simulink model "PVAndBatteryIntegratedPlantForBlackStart"  (R2025b)
settings: Solver=FixedStepAuto  StartTime=0.0  StopTime=tsim  FixedStep=1e-6  RelTol=1e-9  AbsTol=1e-7
InitFcn:
  | %% Black Start Sequence
  | t0 = 0; % Battery IBR initial time
  | t1 = 0.15; % PV IBR initial time
  | t2 = 0.5; % Two IBR sync time
  | t3 = 0.8; % Additional motor load connect
  | t4 = 1.1; % Grid reconnection
  | tsim = 1.5; % Total simulation time
  | 
  | %% initialize
  | Vdc = 400;
  | Vnom = 100;
  | Prated = 10000;
  | Qrated = 0;
  | Srated = sqrt(Prated^2+Qrated^2);
  | wnom = 2*pi*60;
  | fnom = 60;
  | Vminpu = 0.95;
  | 
  | kv = Vnom;
  | ki = 3*Vnom/Srated;
  | 
  | dwmax = 0.5*2*pi;
  | trisemax = 0.1;
  | 
  | C = 1/sqrt(2)/Vminpu^2/dwmax;
  | L = 1/C/wnom^2;
  | tau = C/kv/ki;
  | epsilon = sqrt(L/C);
  | ksy = 3/2/trisemax;
  | 
  | V_voc_1 = 0;
  | V_voc_2 = 0;
  | 
  | % filter
  | Rf = 0.05;
  | Lf = 500e-6;
  | % pwm
  | fsw = 10e3;
  | % simulation
  | Ts = 1e-6;
  | 
  | % load
  | Rl = 3*Vnom^2/Prated;
  | Rl1 = Rl;
  | Rl2 = 2*Rl;
  | Rl3 = 20*Rl;
  | % grid
  | Rg = 0.05;
  | Lg = 50e-6;
  | 
  | % DCDC converter
  | Kp_V = 1;
  | Ki_V = 0.02;
  | Imax = 110;
  | Kp_I = 0.0001;
  | Ki_I = 1;
  | Vcmax = 1;
undefined symbols (not defined in the file): alpha, C_voc, Diode_class, Half_BridgeConverter_class, L_voc, Ll, Mosfet_class, PWMGenerator_DC_DC__class, R_voc, Three_PhaseBreaker_class, Three_PhaseSource_class, Three_PhaseTransformer_2_class, Three_PhaseV_IMeasuremen_class
libraries: nesl_utility x69, ee_lib x49, fl_lib x36, mcbeeMathTransformLib x9, simulink x6, spsParallelRLCBranchLib x3, eePwmGeneratorTwoLevel x2, spsControlledCurrentSourceLib x2, elec_conv_HighZElecRef x2, slpidlib x2, spsSecondOrderFilterLib x1, spsCurrentMeasurementLib x1
(part 4 of 4)

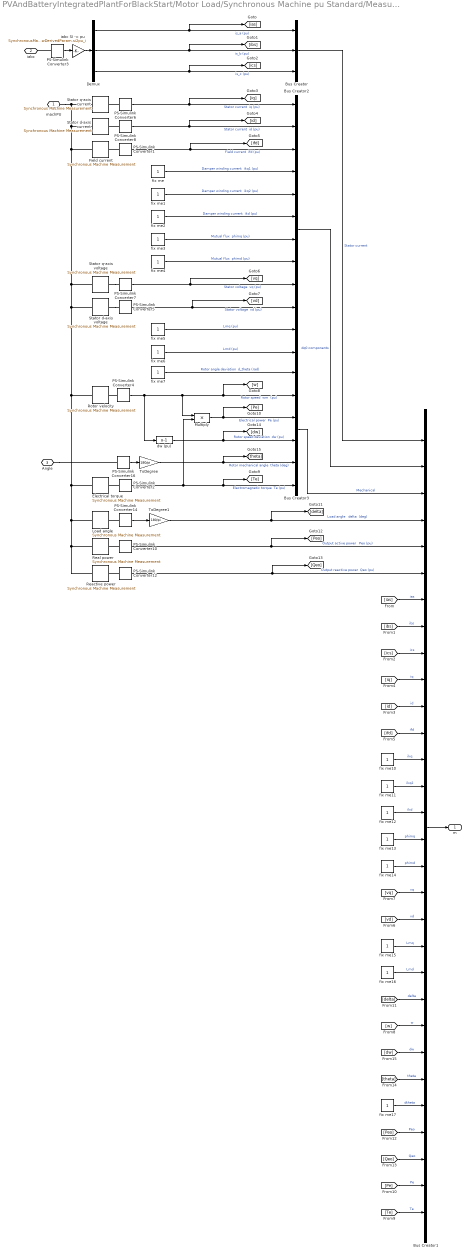
== system PVAndBatteryIntegratedPlantForBlackStart/Motor Load/Synchronous Machine pu Standard/Measurement ==
  Bus Creator : BusCreator  Inputs=3
  Bus Creator1 : BusCreator  Inputs=30
  Bus Creator2 : BusCreator  Inputs=12
  Bus Creator3 : BusCreator  Inputs=6
  Demux : Demux  Outputs=3
  Electrical torque : ee_lib/Electromechanical/Synchronous/Synchronous Machine Measurement  output_idx=3
      settings: InternalSimscapePortConfiguration="{\"Bottom\":[],\"Left\":[{\"id\":\"pu_input\",\"label\":\"pu\",\"type\":\"input\"}],\"Right\":[{\"id\":\"pu_output\",\"label\":\"o\",\"type\":\"output\"}],\"Top\":[]}"
  Field current : ee_lib/Electromechanical/Synchronous/Synchronous Machine Measurement  output_idx=2
      settings: InternalSimscapePortConfiguration="{\"Bottom\":[],\"Left\":[{\"id\":\"pu_input\",\"label\":\"pu\",\"type\":\"input\"}],\"Right\":[{\"id\":\"pu_output\",\"label\":\"o\",\"type\":\"output\"}],\"Top\":[]}"
  Load angle : ee_lib/Electromechanical/Synchronous/Synchronous Machine Measurement  output_idx=18
      settings: InternalSimscapePortConfiguration="{\"Bottom\":[],\"Left\":[{\"id\":\"pu_input\",\"label\":\"pu\",\"type\":\"input\"}],\"Right\":[{\"id\":\"pu_output\",\"label\":\"o\",\"type\":\"output\"}],\"Top\":[]}"
  Multiply : Product
  PS-Simulink Converter{1..8,10,12,14,16} (12 alike) : nesl_utility/PS-Simulink Converter  PhysicalDomain=network_engine_domain  SubClassName=ps_output  LeftPortType=input  RightPortType=output  PseudoPeriodic=off  Frequencies=[]  VectorFormat=1-D array  Unit=1  AffineConversion=off
  Reactive power : ee_lib/Electromechanical/Synchronous/Synchronous Machine Measurement  output_idx=13
      settings: InternalSimscapePortConfiguration="{\"Bottom\":[],\"Left\":[{\"id\":\"pu_input\",\"label\":\"pu\",\"type\":\"input\"}],\"Right\":[{\"id\":\"pu_output\",\"label\":\"o\",\"type\":\"output\"}],\"Top\":[]}"
  Real power : ee_lib/Electromechanical/Synchronous/Synchronous Machine Measurement  output_idx=12
      settings: InternalSimscapePortConfiguration="{\"Bottom\":[],\"Left\":[{\"id\":\"pu_input\",\"label\":\"pu\",\"type\":\"input\"}],\"Right\":[{\"id\":\"pu_output\",\"label\":\"o\",\"type\":\"output\"}],\"Top\":[]}"
  Rotor velocity : ee_lib/Electromechanical/Synchronous/Synchronous Machine Measurement  output_idx=4
      settings: InternalSimscapePortConfiguration="{\"Bottom\":[],\"Left\":[{\"id\":\"pu_input\",\"label\":\"pu\",\"type\":\"input\"}],\"Right\":[{\"id\":\"pu_output\",\"label\":\"o\",\"type\":\"output\"}],\"Top\":[]}"
  Stator d-axis current : ee_lib/Electromechanical/Synchronous/Synchronous Machine Measurement  output_idx=8
      settings: InternalSimscapePortConfiguration="{\"Bottom\":[],\"Left\":[{\"id\":\"pu_input\",\"label\":\"pu\",\"type\":\"input\"}],\"Right\":[{\"id\":\"pu_output\",\"label\":\"o\",\"type\":\"output\"}],\"Top\":[]}"
  Stator d-axis voltage : ee_lib/Electromechanical/Synchronous/Synchronous Machine Measurement  output_idx=5
      settings: InternalSimscapePortConfiguration="{\"Bottom\":[],\"Left\":[{\"id\":\"pu_input\",\"label\":\"pu\",\"type\":\"input\"}],\"Right\":[{\"id\":\"pu_output\",\"label\":\"o\",\"type\":\"output\"}],\"Top\":[]}"
  Stator q-axis current : ee_lib/Electromechanical/Synchronous/Synchronous Machine Measurement  output_idx=9
      settings: InternalSimscapePortConfiguration="{\"Bottom\":[],\"Left\":[{\"id\":\"pu_input\",\"label\":\"pu\",\"type\":\"input\"}],\"Right\":[{\"id\":\"pu_output\",\"label\":\"o\",\"type\":\"output\"}],\"Top\":[]}"
  Stator q-axis voltage : ee_lib/Electromechanical/Synchronous/Synchronous Machine Measurement  output_idx=6
      settings: InternalSimscapePortConfiguration="{\"Bottom\":[],\"Left\":[{\"id\":\"pu_input\",\"label\":\"pu\",\"type\":\"input\"}],\"Right\":[{\"id\":\"pu_output\",\"label\":\"o\",\"type\":\"output\"}],\"Top\":[]}"
  ToDegree : Gain  Gain=180/pi
  ToDegree1 : Gain  Gain=180/pi
  dw (pu) : Bias  Bias=-1  SaturateOnIntegerOverflow=off
  fix me{,1..7,10..17} (16 alike) : Constant
  "iabc SI -> pu" : Gain  Gain=SynchronousMachinePuStan_class('Mechanical power Pm',[6000 122.5 60],[0.1028 0.02056 2],20,[0 0 0 0 0 0 0 0 1],[0.6404 0.7127 0.8441 0.9214 0.9956 1.082 1.19 1.316 1.457;0.7 0.7698 0.8872 0.9466 0.9969 1.046 1.1 1.151 1.201],'on','Salient-pole','Short-circuit','Short-circuit',[1.81 0.3 0.23 1.76 0.65 0.25 0.15],[2.24 0.17 0.12 1.02 0.13 0.08],[4.4849 0.0681 0.1],[8 0.03 1 0.07],[4.49 0.0681 0.0513],[8 0.03 0.3371 0.0295],[1.01 0.053 0.1],[1.3201 0.023 1 0.07],[0.012 0.003 0.003],[1.3201 0.0231 0.3371 0.0295]).objParamMappingDerived.NewDerivedParam.si2pu_i
  machPU : PMIOPort  Side=Left
  iabc : PMIOPort  Port=2  Side=Left
  Angle : PMIOPort  Port=3  Side=Left
  m : Outport  VectorParamsAs1DForOutWhenUnconnected=off
  wires:
  "iabc SI -> pu"/1 -> Demux/1
  PS-Simulink Converter12/1 -> Bus Creator1/6, [Qeo]  "Output reactive power  Qeo (pu)"
  PS-Simulink Converter10/1 -> Bus Creator1/5, [Peo]  "Output active power   Peo (pu)"
  PS-Simulink Converter14/1 -> ToDegree1/1
  PS-Simulink Converter3/1 -> "iabc SI -> pu"/1
  Demux/3 -> [ics], Bus Creator/3  "is_c (pu)"
  Demux/2 -> [ibs], Bus Creator/2  "is_b (pu)"
  Demux/1 -> [ias], Bus Creator/1  "is_a (pu)"
  Bus Creator3/1 -> Bus Creator1/3  "Mechanical"
  Bus Creator2/1 -> Bus Creator1/2  "dq0 components"
  Bus Creator/1 -> Bus Creator1/1  "Stator current"
  Bus Creator1/1 -> m/1
  PS-Simulink Converter8/1 -> [id], Bus Creator2/2  "Stator current  id (pu)"
  PS-Simulink Converter6/1 -> [iq], Bus Creator2/1  "Stator current  iq (pu)"
  PS-Simulink Converter5/1 -> Bus Creator2/10, [vd]  "Stator voltage  vd (pu)"
  PS-Simulink Converter7/1 -> Bus Creator2/9, [vq]  "Stator voltage  vq (pu)"
  PS-Simulink Converter4/1 -> dw (pu)/1, Bus Creator3/2, [w], Multiply/1  "Rotor speed  wm  (pu)"
  PS-Simulink Converter2/1 -> Multiply/2, [Te], Bus Creator3/6  "Electromagnetic torque  Te (pu)"
  PS-Simulink Converter1/1 -> [ifd], Bus Creator2/3  "Field current  ifd (pu)"
  Multiply/1 -> [Pe], Bus Creator3/3  "Electrical power  Pe (pu)"
  [ias] -> Bus Creator1/7  "ias"
  [ibs] -> Bus Creator1/8  "ibs"
  [ics] -> Bus Creator1/9  "ics"
  [ifd] -> Bus Creator1/12  "ifd"
  fix me6/1 -> Bus Creator2/12  "Lmd (pu)"
  fix me5/1 -> Bus Creator2/11  "Lmq (pu)"
  fix me7/1 -> Bus Creator3/1  "Rotor angle deviation  d_theta (rad)"
  dw (pu)/1 -> [dw], Bus Creator3/4  "Rotor speed deviation  dw (pu)"
  ToDegree/1 -> [theta], Bus Creator3/5  "Rotor mechanical angle  theta (deg)"
  PS-Simulink Converter16/1 -> ToDegree/1
  ToDegree1/1 -> Bus Creator1/4, [delta]  "Load angle   delta  (deg)"
  [id] -> Bus Creator1/11  "id"
  [iq] -> Bus Creator1/10  "iq"
  fix me10/1 -> Bus Creator1/13  "ikq"
  fix me11/1 -> Bus Creator1/14  "ikq2"
  fix me12/1 -> Bus Creator1/15  "ikd"
  fix me13/1 -> Bus Creator1/16  "phimq"
  fix me14/1 -> Bus Creator1/17  "phimd"
  [vq] -> Bus Creator1/18  "vq"
  [vd] -> Bus Creator1/19  "vd"
  fix me16/1 -> Bus Creator1/21  "Lmd"
  fix me15/1 -> Bus Creator1/20  "Lmq"
  [delta] -> Bus Creator1/22  "delta"
  [w] -> Bus Creator1/23  "w"
  [dw] -> Bus Creator1/24  "dw"
  [theta] -> Bus Creator1/25  "theta"
  fix me17/1 -> Bus Creator1/26  "dtheta"
  [Peo] -> Bus Creator1/27  "Peo"
  [Qeo] -> Bus Creator1/28  "Qeo"
  [Pe] -> Bus Creator1/29  "Pe"
  [Te] -> Bus Creator1/30  "Te"
  fix me/1 -> Bus Creator2/4  "Damper winding current  ikq1 (pu)"
  fix me1/1 -> Bus Creator2/5  "Damper winding current  ikq2 (pu)"
  fix me2/1 -> Bus Creator2/6  "Damper winding current  ikd (pu)"
  fix me3/1 -> Bus Creator2/7  "Mutual flux  phimq (pu)"
  fix me4/1 -> Bus Creator2/8  "Mutual flux  phimd (pu)"
  connections:
  PS-Simulink Converter3/LConn1 -- iabc/RConn1
  Stator q-axis current/LConn1 -- Stator d-axis voltage/LConn1 -- Reactive power/LConn1 -- Real power/LConn1 -- Load angle/LConn1 -- Electrical torque/LConn1 -- Rotor velocity/LConn1 -- Stator q-axis voltage/LConn1 -- Field current/LConn1 -- Stator d-axis current/LConn1 -- machPU/RConn1
  PS-Simulink Converter14/LConn1 -- Load angle/RConn1
  PS-Simulink Converter12/LConn1 -- Reactive power/RConn1
  PS-Simulink Converter10/LConn1 -- Real power/RConn1
  PS-Simulink Converter8/LConn1 -- Stator d-axis current/RConn1
  Stator d-axis voltage/RConn1 -- PS-Simulink Converter5/LConn1
  PS-Simulink Converter6/LConn1 -- Stator q-axis current/RConn1
  Stator q-axis voltage/RConn1 -- PS-Simulink Converter7/LConn1
  PS-Simulink Converter4/LConn1 -- Rotor velocity/RConn1
  PS-Simulink Converter2/LConn1 -- Electrical torque/RConn1
  PS-Simulink Converter1/LConn1 -- Field current/RConn1
  Angle/RConn1 -- PS-Simulink Converter16/LConn1

== system PVAndBatteryIntegratedPlantForBlackStart/PV Inverter /Inverter/Half-Bridge Converter ==
  " g " : Inport
  BL : Inport  Port=2
  Compare To Constant : simulink/Logic and Bit Operations/Compare To Constant  relop=<=  const=0.5  OutDataTypeStr=boolean
  Data Type Conversion : DataTypeConversion  OutDataTypeStr=double  SaturateOnIntegerOverflow=off  RndMeth=Floor
  Demux : Demux  Outputs=2
  Multiply : Product
  Simulink-PS Converter : nesl_utility/Simulink-PS Converter  PhysicalDomain=network_engine_domain  SubClassName=ps_input  LeftPortType=input  RightPortType=output  PseudoPeriodic=off  Frequencies=[]  NoiseDistribution=none  NoiseParameters=[]  Unit=1  AffineConversion=off  FilteringAndDerivatives=provide  SimscapeFilterOrder=1  InputFilterTimeConstant=0.001  UdotUserProvided=0
  Simulink-PS Converter1 : nesl_utility/Simulink-PS Converter  PhysicalDomain=network_engine_domain  SubClassName=ps_input  LeftPortType=input  RightPortType=output  PseudoPeriodic=off  Frequencies=[]  NoiseDistribution=none  NoiseParameters=[]  Unit=1  AffineConversion=off  FilteringAndDerivatives=provide  SimscapeFilterOrder=1  InputFilterTimeConstant=0.001  UdotUserProvided=0
  Two-Pulse Gate Multiplexer : ee_lib/Semiconductors & Converters/Converters/Two-Pulse Gate Multiplexer  port_option=ee.enum.controlport.ps
      settings: InternalSimscapePortConfiguration="{\"Bottom\":[],\"Left\":[{\"id\":\"G1_ps\",\"label\":\"G1\",\"type\":\"input\"},{\"id\":\"G2_ps\",\"label\":\"G2\",\"type\":\"input\"}],\"Right\":[{\"id\":\"p\",\"label\":\"G\",\"type\":\"foundation.electrical.four_phase\"}],\"Top\":[]}"
  Two-Quadrant Chopper : ee_lib/Semiconductors & Converters/Converters/Two-Quadrant Chopper  device_type=3  Vf=Half_BridgeConverter_class('Switching devices',0.001,1000000,Inf,0.001,1000000,Inf,0.001).objParamMappingDerived.NewDerivedParam.Vf V  Ron=Half_BridgeConverter_class('Switching devices',0.001,1000000,Inf,0.001,1000000,Inf,0.001).objParamMappingDerived.NewDerivedParam.Ron Ohm  Rds=0.001 Ohm  Goff=Half_BridgeConverter_class('Switching devices',0.001,1000000,Inf,0.001,1000000,Inf,0.001).objParamMappingDerived.NewDerivedParam.Goff 1/Ohm  Vgt=1 V  Vgt_off=-1 V  Ih=1 A  Vth=0.5 V  K=0  diode_param=2  diode_Vf=Half_BridgeConverter_class('Switching devices',0.001,1000000,Inf,0.001,1000000,Inf,0.001).objParamMappingDerived.NewDerivedParam.diode_Vf V  diode_Ron=Half_BridgeConverter_class('Switching devices',0.001,1000000,Inf,0.001,1000000,Inf,0.001).objParamMappingDerived.NewDerivedParam.diode_Ron Ohm  diode_Goff=Half_BridgeConverter_class('Switching devices',0.001,1000000,Inf,0.001,1000000,Inf,0.001).objParamMappingDerived.NewDerivedParam.diode_Goff 1/Ohm  diode_C=50 nF  diode_iRM=-235 A  diode_iF=300 A  diode_idot=-50 A/us  diode_trr_param=1  diode_trr_factor=3  diode_trr=15 us  diode_Qrr=1500 s*uA  snubber_type=0  Cs=Half_BridgeConverter_class('Switching devices',0.001,1000000,Inf,0.001,1000000,Inf,0.001).objParamMappingDerived.NewDerivedParam.Cs F  Rs=Half_BridgeConverter_class('Switching devices',0.001,1000000,Inf,0.001,1000000,Inf,0.001).objParamMappingDerived.NewDerivedParam.Rs Ohm
      settings: InternalSimscapePortConfiguration="{\"Bottom\":[],\"Left\":[{\"id\":\"G\",\"label\":\"G\",\"type\":\"foundation.electrical.four_phase\"},{\"id\":\"p1\",\"label\":\"1+\",\"type\":\"foundation.electrical.electrical\"},{\"id\":\"n1\",\"label\":\"1-\",\"type\":\"foundation.electrical.electrical\"}],\"Right\":[{\"id\":\"p2\",\"label\":\"2+\",\"type\":\"foundation.electrical.electrical\"},{\"id\":\"n2\",\"label\":\"2-\",\"type\":\"foundation.electrical.electrical\"}],\"Top\":[]}"
  + : PMIOPort  Side=Right
  - : PMIOPort  Port=2  Side=Right
  1 : PMIOPort  Port=3  Side=Left
  wires:
  Demux/2 -> Simulink-PS Converter1/1
  Demux/1 -> Simulink-PS Converter/1
  Multiply/1 -> Demux/1
  Data Type Conversion/1 -> Multiply/2
  Compare To Constant/1 -> Data Type Conversion/1
  BL/1 -> Compare To Constant/1
  " g "/1 -> Multiply/1
  connections:
  Simulink-PS Converter1/RConn1 -- Two-Pulse Gate Multiplexer/LConn2
  Two-Pulse Gate Multiplexer/RConn1 -- Two-Quadrant Chopper/LConn1
  Simulink-PS Converter/RConn1 -- Two-Pulse Gate Multiplexer/LConn1
  +/RConn1 -- Two-Quadrant Chopper/LConn2
  1/RConn1 -- Two-Quadrant Chopper/RConn1
  Two-Quadrant Chopper/LConn3 -- Two-Quadrant Chopper/RConn2 -- -/RConn1

== system PVAndBatteryIntegratedPlantForBlackStart/PV Inverter /Inverter/Half-Bridge Converter1 ==
  " g " : Inport
  BL : Inport  Port=2
  Compare To Constant : simulink/Logic and Bit Operations/Compare To Constant  relop=<=  const=0.5  OutDataTypeStr=boolean
  Data Type Conversion : DataTypeConversion  OutDataTypeStr=double  SaturateOnIntegerOverflow=off  RndMeth=Floor
  Demux : Demux  Outputs=2
  Multiply : Product
  Simulink-PS Converter : nesl_utility/Simulink-PS Converter  PhysicalDomain=network_engine_domain  SubClassName=ps_input  LeftPortType=input  RightPortType=output  PseudoPeriodic=off  Frequencies=[]  NoiseDistribution=none  NoiseParameters=[]  Unit=1  AffineConversion=off  FilteringAndDerivatives=provide  SimscapeFilterOrder=1  InputFilterTimeConstant=0.001  UdotUserProvided=0
  Simulink-PS Converter1 : nesl_utility/Simulink-PS Converter  PhysicalDomain=network_engine_domain  SubClassName=ps_input  LeftPortType=input  RightPortType=output  PseudoPeriodic=off  Frequencies=[]  NoiseDistribution=none  NoiseParameters=[]  Unit=1  AffineConversion=off  FilteringAndDerivatives=provide  SimscapeFilterOrder=1  InputFilterTimeConstant=0.001  UdotUserProvided=0
  Two-Pulse Gate Multiplexer : ee_lib/Semiconductors & Converters/Converters/Two-Pulse Gate Multiplexer  port_option=ee.enum.controlport.ps
      settings: InternalSimscapePortConfiguration="{\"Bottom\":[],\"Left\":[{\"id\":\"G1_ps\",\"label\":\"G1\",\"type\":\"input\"},{\"id\":\"G2_ps\",\"label\":\"G2\",\"type\":\"input\"}],\"Right\":[{\"id\":\"p\",\"label\":\"G\",\"type\":\"foundation.electrical.four_phase\"}],\"Top\":[]}"
  Two-Quadrant Chopper : ee_lib/Semiconductors & Converters/Converters/Two-Quadrant Chopper  device_type=3  Vf=Half_BridgeConverter_class('Switching devices',0.001,1000000,Inf,0.001,1000000,Inf,0.001).objParamMappingDerived.NewDerivedParam.Vf V  Ron=Half_BridgeConverter_class('Switching devices',0.001,1000000,Inf,0.001,1000000,Inf,0.001).objParamMappingDerived.NewDerivedParam.Ron Ohm  Rds=0.001 Ohm  Goff=Half_BridgeConverter_class('Switching devices',0.001,1000000,Inf,0.001,1000000,Inf,0.001).objParamMappingDerived.NewDerivedParam.Goff 1/Ohm  Vgt=1 V  Vgt_off=-1 V  Ih=1 A  Vth=0.5 V  K=0  diode_param=2  diode_Vf=Half_BridgeConverter_class('Switching devices',0.001,1000000,Inf,0.001,1000000,Inf,0.001).objParamMappingDerived.NewDerivedParam.diode_Vf V  diode_Ron=Half_BridgeConverter_class('Switching devices',0.001,1000000,Inf,0.001,1000000,Inf,0.001).objParamMappingDerived.NewDerivedParam.diode_Ron Ohm  diode_Goff=Half_BridgeConverter_class('Switching devices',0.001,1000000,Inf,0.001,1000000,Inf,0.001).objParamMappingDerived.NewDerivedParam.diode_Goff 1/Ohm  diode_C=50 nF  diode_iRM=-235 A  diode_iF=300 A  diode_idot=-50 A/us  diode_trr_param=1  diode_trr_factor=3  diode_trr=15 us  diode_Qrr=1500 s*uA  snubber_type=0  Cs=Half_BridgeConverter_class('Switching devices',0.001,1000000,Inf,0.001,1000000,Inf,0.001).objParamMappingDerived.NewDerivedParam.Cs F  Rs=Half_BridgeConverter_class('Switching devices',0.001,1000000,Inf,0.001,1000000,Inf,0.001).objParamMappingDerived.NewDerivedParam.Rs Ohm
      settings: InternalSimscapePortConfiguration="{\"Bottom\":[],\"Left\":[{\"id\":\"G\",\"label\":\"G\",\"type\":\"foundation.electrical.four_phase\"},{\"id\":\"p1\",\"label\":\"1+\",\"type\":\"foundation.electrical.electrical\"},{\"id\":\"n1\",\"label\":\"1-\",\"type\":\"foundation.electrical.electrical\"}],\"Right\":[{\"id\":\"p2\",\"label\":\"2+\",\"type\":\"foundation.electrical.electrical\"},{\"id\":\"n2\",\"label\":\"2-\",\"type\":\"foundation.electrical.electrical\"}],\"Top\":[]}"
  + : PMIOPort  Side=Right
  - : PMIOPort  Port=2  Side=Right
  1 : PMIOPort  Port=3  Side=Left
  wires:
  Demux/2 -> Simulink-PS Converter1/1
  Demux/1 -> Simulink-PS Converter/1
  Multiply/1 -> Demux/1
  Data Type Conversion/1 -> Multiply/2
  Compare To Constant/1 -> Data Type Conversion/1
  BL/1 -> Compare To Constant/1
  " g "/1 -> Multiply/1
  connections:
  Simulink-PS Converter1/RConn1 -- Two-Pulse Gate Multiplexer/LConn2
  Two-Pulse Gate Multiplexer/RConn1 -- Two-Quadrant Chopper/LConn1
  Simulink-PS Converter/RConn1 -- Two-Pulse Gate Multiplexer/LConn1
  +/RConn1 -- Two-Quadrant Chopper/LConn2
  1/RConn1 -- Two-Quadrant Chopper/RConn1
  Two-Quadrant Chopper/LConn3 -- Two-Quadrant Chopper/RConn2 -- -/RConn1

== system PVAndBatteryIntegratedPlantForBlackStart/PV Inverter /Inverter/Half-Bridge Converter2 ==
  " g " : Inport
  BL : Inport  Port=2
  Compare To Constant : simulink/Logic and Bit Operations/Compare To Constant  relop=<=  const=0.5  OutDataTypeStr=boolean
  Data Type Conversion : DataTypeConversion  OutDataTypeStr=double  SaturateOnIntegerOverflow=off  RndMeth=Floor
  Demux : Demux  Outputs=2
  Multiply : Product
  Simulink-PS Converter : nesl_utility/Simulink-PS Converter  PhysicalDomain=network_engine_domain  SubClassName=ps_input  LeftPortType=input  RightPortType=output  PseudoPeriodic=off  Frequencies=[]  NoiseDistribution=none  NoiseParameters=[]  Unit=1  AffineConversion=off  FilteringAndDerivatives=provide  SimscapeFilterOrder=1  InputFilterTimeConstant=0.001  UdotUserProvided=0
  Simulink-PS Converter1 : nesl_utility/Simulink-PS Converter  PhysicalDomain=network_engine_domain  SubClassName=ps_input  LeftPortType=input  RightPortType=output  PseudoPeriodic=off  Frequencies=[]  NoiseDistribution=none  NoiseParameters=[]  Unit=1  AffineConversion=off  FilteringAndDerivatives=provide  SimscapeFilterOrder=1  InputFilterTimeConstant=0.001  UdotUserProvided=0
  Two-Pulse Gate Multiplexer : ee_lib/Semiconductors & Converters/Converters/Two-Pulse Gate Multiplexer  port_option=ee.enum.controlport.ps
      settings: InternalSimscapePortConfiguration="{\"Bottom\":[],\"Left\":[{\"id\":\"G1_ps\",\"label\":\"G1\",\"type\":\"input\"},{\"id\":\"G2_ps\",\"label\":\"G2\",\"type\":\"input\"}],\"Right\":[{\"id\":\"p\",\"label\":\"G\",\"type\":\"foundation.electrical.four_phase\"}],\"Top\":[]}"
  Two-Quadrant Chopper : ee_lib/Semiconductors & Converters/Converters/Two-Quadrant Chopper  device_type=3  Vf=Half_BridgeConverter_class('Switching devices',0.001,1000000,Inf,0.001,1000000,Inf,0.001).objParamMappingDerived.NewDerivedParam.Vf V  Ron=Half_BridgeConverter_class('Switching devices',0.001,1000000,Inf,0.001,1000000,Inf,0.001).objParamMappingDerived.NewDerivedParam.Ron Ohm  Rds=0.001 Ohm  Goff=Half_BridgeConverter_class('Switching devices',0.001,1000000,Inf,0.001,1000000,Inf,0.001).objParamMappingDerived.NewDerivedParam.Goff 1/Ohm  Vgt=1 V  Vgt_off=-1 V  Ih=1 A  Vth=0.5 V  K=0  diode_param=2  diode_Vf=Half_BridgeConverter_class('Switching devices',0.001,1000000,Inf,0.001,1000000,Inf,0.001).objParamMappingDerived.NewDerivedParam.diode_Vf V  diode_Ron=Half_BridgeConverter_class('Switching devices',0.001,1000000,Inf,0.001,1000000,Inf,0.001).objParamMappingDerived.NewDerivedParam.diode_Ron Ohm  diode_Goff=Half_BridgeConverter_class('Switching devices',0.001,1000000,Inf,0.001,1000000,Inf,0.001).objParamMappingDerived.NewDerivedParam.diode_Goff 1/Ohm  diode_C=50 nF  diode_iRM=-235 A  diode_iF=300 A  diode_idot=-50 A/us  diode_trr_param=1  diode_trr_factor=3  diode_trr=15 us  diode_Qrr=1500 s*uA  snubber_type=0  Cs=Half_BridgeConverter_class('Switching devices',0.001,1000000,Inf,0.001,1000000,Inf,0.001).objParamMappingDerived.NewDerivedParam.Cs F  Rs=Half_BridgeConverter_class('Switching devices',0.001,1000000,Inf,0.001,1000000,Inf,0.001).objParamMappingDerived.NewDerivedParam.Rs Ohm
      settings: InternalSimscapePortConfiguration="{\"Bottom\":[],\"Left\":[{\"id\":\"G\",\"label\":\"G\",\"type\":\"foundation.electrical.four_phase\"},{\"id\":\"p1\",\"label\":\"1+\",\"type\":\"foundation.electrical.electrical\"},{\"id\":\"n1\",\"label\":\"1-\",\"type\":\"foundation.electrical.electrical\"}],\"Right\":[{\"id\":\"p2\",\"label\":\"2+\",\"type\":\"foundation.electrical.electrical\"},{\"id\":\"n2\",\"label\":\"2-\",\"type\":\"foundation.electrical.electrical\"}],\"Top\":[]}"
  + : PMIOPort  Side=Right
  - : PMIOPort  Port=2  Side=Right
  1 : PMIOPort  Port=3  Side=Left
  wires:
  Demux/2 -> Simulink-PS Converter1/1
  Demux/1 -> Simulink-PS Converter/1
  Multiply/1 -> Demux/1
  Data Type Conversion/1 -> Multiply/2
  Compare To Constant/1 -> Data Type Conversion/1
  BL/1 -> Compare To Constant/1
  " g "/1 -> Multiply/1
  connections:
  Simulink-PS Converter1/RConn1 -- Two-Pulse Gate Multiplexer/LConn2
  Two-Pulse Gate Multiplexer/RConn1 -- Two-Quadrant Chopper/LConn1
  Simulink-PS Converter/RConn1 -- Two-Pulse Gate Multiplexer/LConn1
  +/RConn1 -- Two-Quadrant Chopper/LConn2
  1/RConn1 -- Two-Quadrant Chopper/RConn1
  Two-Quadrant Chopper/LConn3 -- Two-Quadrant Chopper/RConn2 -- -/RConn1

== system PVAndBatteryIntegratedPlantForBlackStart/PV Inverter /Three-Phase Breaker/com ==
  AND : Logic  Operator=NXOR  Inputs=5  IconShape=distinctive  AllPortsSameDT=off  OutDataTypeStr=boolean
  Data Type Conversion : DataTypeConversion  SaturateOnIntegerOverflow=off  RndMeth=Floor
  Simulink-PS Converter : nesl_utility/Simulink-PS Converter  PhysicalDomain=network_engine_domain  SubClassName=ps_input  LeftPortType=input  RightPortType=output  PseudoPeriodic=off  Frequencies=[]  NoiseDistribution=none  NoiseParameters=[]  Unit=1  AffineConversion=off  FilteringAndDerivatives=provide  SimscapeFilterOrder=1  InputFilterTimeConstant=0.001  UdotUserProvided=0
  Step : Step  Time=Three_PhaseBreaker_class('open',1000000,Inf,t1,'off').objParamMappingDerived.NewDerivedParam.switchTime1  SampleTime=0
  Step1 : Step  Time=Three_PhaseBreaker_class('open',1000000,Inf,t1,'off').objParamMappingDerived.NewDerivedParam.switchTime2  SampleTime=0
  Step2 : Step  Time=Three_PhaseBreaker_class('open',1000000,Inf,t1,'off').objParamMappingDerived.NewDerivedParam.switchTime3  SampleTime=0
  Step3 : Step  Time=Three_PhaseBreaker_class('open',1000000,Inf,t1,'off').objParamMappingDerived.NewDerivedParam.switchTime4  SampleTime=0
  Step4 : Step  Time=Three_PhaseBreaker_class('open',1000000,Inf,t1,'off').objParamMappingDerived.NewDerivedParam.switchTime5  SampleTime=0
  CB : PMIOPort  Side=Right
  wires:
  Data Type Conversion/1 -> Simulink-PS Converter/1
  Step4/1 -> AND/5
  AND/1 -> Data Type Conversion/1
  Step3/1 -> AND/4
  Step1/1 -> AND/2
  Step/1 -> AND/1
  Step2/1 -> AND/3
  connections:
  Simulink-PS Converter/RConn1 -- CB/RConn1

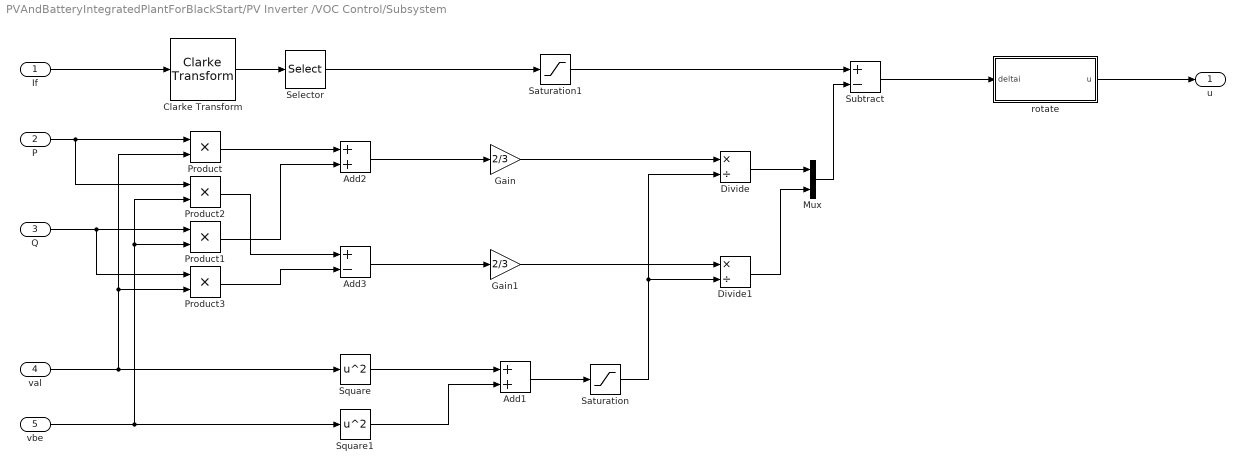
== system PVAndBatteryIntegratedPlantForBlackStart/PV Inverter /VOC Control/Subsystem ==
  If : Inport
  P : Inport  Port=2
  Q : Inport  Port=3
  val : Inport  Port=4
  vbe : Inport  Port=5
  Add1 : Sum
  Add2 : Sum
  Add3 : Sum  Inputs=+-
  Clarke Transform : mcbeeMathTransformLib/Clarke Transform  PowerInvariant=off  UseWithEmbedded=off  PhaseInput=Two inputs
      settings: LibrarySourceBlock=|
      | ee_sl_lib/Mathematical
      | Transforms/Clarke Transform
  Divide : Product  Inputs=*/
  Divide1 : Product  Inputs=*/
  Gain : Gain  Gain=2/3
  Gain1 : Gain  Gain=2/3
  Mux : Mux  Inputs=2
  Product{,1..3} (4 alike) : Product
  Saturation : Saturate  UpperLimit=inf  LowerLimit=1e-9
  Saturation1 : Saturate  UpperLimit=1e3  LowerLimit=-1e3
  Selector : Selector  InputPortWidth=3  IndexOptions=Index vector (dialog)  Indices=[1 2]  OutputSizes=1
  Square : Math  Operator=square
  Square1 : Math  Operator=square
  Subtract : Sum  Inputs=+-
  rotate : Subsystem
  u : Outport
  wires:
  rotate/1(u) -> u/1
  Subtract/1 -> rotate/1(deltai)
  Mux/1 -> Subtract/2
  Divide1/1 -> Mux/2
  Divide/1 -> Mux/1
  Gain1/1 -> Divide1/1
  Add3/1 -> Gain1/1
  Product3/1 -> Add3/2
  Product2/1 -> Add3/1
  Saturation/1 -> Divide1/2, Divide/2
  Gain/1 -> Divide/1
  Add2/1 -> Gain/1
  Product1/1 -> Add2/2
  Product/1 -> Add2/1
  Q/1 -> Product1/1, Product3/1
  P/1 -> Product/1, Product2/1
  Add1/1 -> Saturation/1
  Square1/1 -> Add1/2
  Square/1 -> Add1/1
  vbe/1 -> Square1/1, Product1/2, Product2/2
  val/1 -> Square/1, Product/2, Product3/2
  If/1 -> Clarke Transform/1
  Clarke Transform/1 -> Selector/1
  Selector/1 -> Saturation1/1
  Saturation1/1 -> Subtract/1

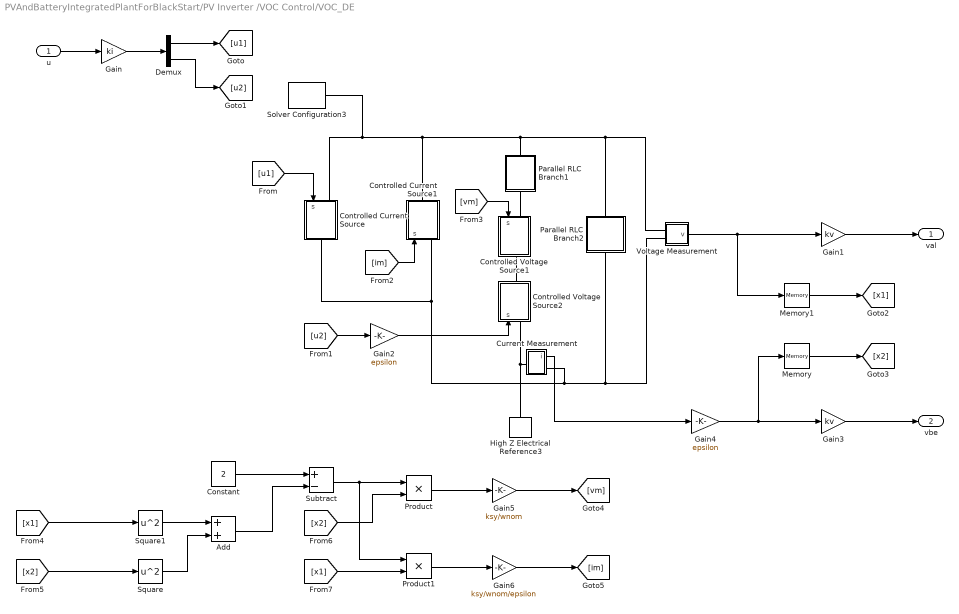
== system PVAndBatteryIntegratedPlantForBlackStart/PV Inverter /VOC Control/VOC_DE ==
  u : Inport
  Add : Sum
  Constant : Constant  Value=2
  Controlled Current Source : Subsystem
      settings: OpenFcn=elec.conv.unmask(gcb);
  Controlled Current Source1 : Subsystem
      settings: OpenFcn=elec.conv.unmask(gcb);
  Controlled Voltage Source1 : Subsystem
      settings: OpenFcn=elec.conv.unmask(gcb);
  Controlled Voltage Source2 : Subsystem
      settings: OpenFcn=elec.conv.unmask(gcb);
  Current Measurement : Subsystem
      settings: OpenFcn=elec.conv.unmask(gcb);
  Demux : Demux  Outputs=2
  Gain : Gain  Gain=ki
  Gain1 : Gain  Gain=kv
  Gain2 : Gain  Gain=epsilon
  Gain3 : Gain  Gain=kv
  Gain4 : Gain  Gain=epsilon
  Gain5 : Gain  Gain=ksy/wnom
  Gain6 : Gain  Gain=ksy/wnom/epsilon
  High Z Electrical Reference3 : elec_conv_HighZElecRef/High Z Electrical Reference  SystemSampleTime=-1  VariantActivationTime=update diagram  EmptyChoice=off  PassThrough=off  PassThroughVariantControl=(default)  EmptyChoiceVariantControl=(default)  AllowFlexibleInterface=on  Latency=0  AutoFrameSizeCalculation=off
  Memory : Memory
  Memory1 : Memory
  Parallel RLC Branch1 : Subsystem
      settings: AttributesFormatString=\n  OpenFcn=elec.conv.unmask(gcb);
  Parallel RLC Branch2 : Subsystem
      settings: AttributesFormatString=\n  OpenFcn=elec.conv.unmask(gcb);
  Product : Product
  Product1 : Product
  Solver Configuration3 : nesl_utility/Solver Configuration  PhysicalDomain=network_engine_domain  SubClassName=solver  LeftPortType=input  RightPortType=generic  Tones=[]  Harmonics=[]  SimulateNoise=off  Profile=off  UseLocalSampling=off  EnableSwitchedLinearOptims=on  FrequencyDomain=off  UseCCode=off  RelTol=0.001  AbsTol=0.001  MinStep=1e-09  ToWorkspace=off  RevertToSquareIcSolve=off  NumHomotopyIterations=100  PhasorMode=off  PhasorModeNumHarmonics=1  ConsistencySolver=NEWTON_XTOL_AFTER_FTOL  IndexReductionMethod=DerivativeReplacement  DoDC=off  ResidualTolerance=1e-09  ConsistencyTolSource=GLOBAL  ConsistencyAbsTol=0.001  ConsistencyRelTol=0.001  ConsistencyTolFactor=0.001  UseLocalSolver=off  LocalSolverChoice=NE_BACKWARD_EULER_ADVANCER  ResolveIndetEquations=on  FunctionEvalNumThread=1  LocalSolverSampleTime=1e-6  DoFixedCost=on  MaxNonlinIter=3  MaxModeIter=2  ComputeImpulses=off  ImpulseIterations=2  LinearAlgebra=auto  LinearAlgebraNumThread=0  EquationFormulation=NE_TIME_EF  DelaysMemoryBudget=1024  AutomaticFiltering=on  FilteringTimeConstant=0.001  PartitionStorageMethod=AS_NEEDED  PartitionMemoryBudget=1024  PartitionMethod=ROBUST  MultibodyUseLocalSolver=off  MultibodyLocalSolverChoice=ODE1  MultibodyLocalSolverSampleTime=0.001
  Square : Math  Operator=square
  Square1 : Math  Operator=square
  Subtract : Sum  Inputs=+-
  Voltage Measurement : Subsystem
      settings: OpenFcn=elec.conv.unmask(gcb);
  val : Outport
  vbe : Outport  Port=2
  wires:
  Gain6/1 -> [im]
  Product1/1 -> Gain6/1
  [x1] -> Product1/2
  Gain5/1 -> [vm]
  Product/1 -> Gain5/1
  [x2] -> Product/2
  Subtract/1 -> Product/1, Product1/1
  Add/1 -> Subtract/2
  Square/1 -> Add/2
  Square1/1 -> Add/1
  Constant/1 -> Subtract/1
  Current Measurement/1(i) -> Gain4/1
  Gain4/1 -> Memory/1, Gain3/1
  Gain3/1 -> vbe/1
  [vm] -> Controlled Voltage Source1/1(s)
  [im] -> Controlled Current Source1/1(s)
  Gain2/1 -> Controlled Voltage Source2/1(s)
  [u2] -> Gain2/1
  [u1] -> Controlled Current Source/1(s)
  Demux/2 -> [u2]
  Demux/1 -> [u1]
  Gain/1 -> Demux/1
  Gain1/1 -> val/1
  Voltage Measurement/1(v) -> Memory1/1, Gain1/1
  u/1 -> Gain/1
  [x1] -> Square1/1
  [x2] -> Square/1
  Memory/1 -> [x2]
  Memory1/1 -> [x1]
  connections:
  Controlled Voltage Source2/LConn1 -- Current Measurement/LConn1 -- High Z Electrical Reference3/LConn1
  Controlled Voltage Source2/RConn1 -- Controlled Voltage Source1/RConn1
  Controlled Voltage Source1/LConn1 -- Parallel RLC Branch1/RConn1
  Voltage Measurement/LConn1 -- Parallel RLC Branch2/LConn1 -- Parallel RLC Branch1/LConn1 -- Controlled Current Source1/RConn1 -- Controlled Current Source/LConn1 -- Solver Configuration3/RConn1
  Voltage Measurement/LConn2 -- Parallel RLC Branch2/RConn1 -- Controlled Current Source/RConn1 -- Controlled Current Source1/LConn1 -- Current Measurement/RConn1

== system PVAndBatteryIntegratedPlantForBlackStart/Battery Inverter/VOC Control/Subsystem/rotate ==
  deltai : Inport
  Demux : Demux  Outputs=2
  Gain : Gain  Gain=-1
  Mux : Mux  Inputs=2
  u : Outport
  wires:
  deltai/1 -> Demux/1
  Mux/1 -> u/1
  Demux/2 -> Gain/1
  Gain/1 -> Mux/1
  Demux/1 -> Mux/2

== system PVAndBatteryIntegratedPlantForBlackStart/Battery Inverter/VOC Control/VOC/f(vc) ==
  vc : Inport
  Gain : Gain  Gain=alpha
  Product : Product  Inputs=3
  f(vc) : Outport
  wires:
  vc/1 -> Product/2, Product/3, Product/1
  Gain/1 -> f(vc)/1
  Product/1 -> Gain/1

== system PVAndBatteryIntegratedPlantForBlackStart/Battery Inverter/VOC Control/VOC_DE/Controlled Current Source ==
  s : Inport
  Controlled Current Source : fl_lib/Electrical/Electrical Sources/Controlled Current Source
  Simulink-PS Converter : nesl_utility/Simulink-PS Converter  PhysicalDomain=network_engine_domain  SubClassName=ps_input  LeftPortType=input  RightPortType=output  PseudoPeriodic=off  Frequencies=[]  NoiseDistribution=none  NoiseParameters=[]  Unit=1  AffineConversion=off  FilteringAndDerivatives=provide  SimscapeFilterOrder=1  InputFilterTimeConstant=0.001  UdotUserProvided=0
  - : PMIOPort  Side=Left
  + : PMIOPort  Port=2  Side=Right
  wires:
  s/1 -> Simulink-PS Converter/1
  connections:
  Simulink-PS Converter/RConn1 -- Controlled Current Source/RConn1
  Controlled Current Source/RConn2 -- -/RConn1
  Controlled Current Source/LConn1 -- +/RConn1

== system PVAndBatteryIntegratedPlantForBlackStart/Battery Inverter/VOC Control/VOC_DE/Controlled Current Source1 ==
  s : Inport
  Controlled Current Source : fl_lib/Electrical/Electrical Sources/Controlled Current Source
  Simulink-PS Converter : nesl_utility/Simulink-PS Converter  PhysicalDomain=network_engine_domain  SubClassName=ps_input  LeftPortType=input  RightPortType=output  PseudoPeriodic=off  Frequencies=[]  NoiseDistribution=none  NoiseParameters=[]  Unit=1  AffineConversion=off  FilteringAndDerivatives=provide  SimscapeFilterOrder=1  InputFilterTimeConstant=0.001  UdotUserProvided=0
  - : PMIOPort  Side=Left
  + : PMIOPort  Port=2  Side=Right
  wires:
  s/1 -> Simulink-PS Converter/1
  connections:
  Simulink-PS Converter/RConn1 -- Controlled Current Source/RConn1
  Controlled Current Source/RConn2 -- -/RConn1
  Controlled Current Source/LConn1 -- +/RConn1

== system PVAndBatteryIntegratedPlantForBlackStart/Battery Inverter/VOC Control/VOC_DE/Controlled Voltage Source1 ==
  s : Inport
  Controlled Voltage Source : fl_lib/Electrical/Electrical Sources/Controlled Voltage Source
  Simulink-PS Converter : nesl_utility/Simulink-PS Converter  PhysicalDomain=network_engine_domain  SubClassName=ps_input  LeftPortType=input  RightPortType=output  PseudoPeriodic=off  Frequencies=[]  NoiseDistribution=none  NoiseParameters=[]  Unit=1  AffineConversion=off  FilteringAndDerivatives=provide  SimscapeFilterOrder=1  InputFilterTimeConstant=0.001  UdotUserProvided=0
  - : PMIOPort  Side=Left
  + : PMIOPort  Port=2  Side=Right
  wires:
  s/1 -> Simulink-PS Converter/1
  connections:
  -/RConn1 -- Controlled Voltage Source/RConn2
  Simulink-PS Converter/RConn1 -- Controlled Voltage Source/RConn1
  Controlled Voltage Source/LConn1 -- +/RConn1

== system PVAndBatteryIntegratedPlantForBlackStart/Battery Inverter/VOC Control/VOC_DE/Controlled Voltage Source2 ==
  s : Inport
  Controlled Voltage Source : fl_lib/Electrical/Electrical Sources/Controlled Voltage Source
  Simulink-PS Converter : nesl_utility/Simulink-PS Converter  PhysicalDomain=network_engine_domain  SubClassName=ps_input  LeftPortType=input  RightPortType=output  PseudoPeriodic=off  Frequencies=[]  NoiseDistribution=none  NoiseParameters=[]  Unit=1  AffineConversion=off  FilteringAndDerivatives=provide  SimscapeFilterOrder=1  InputFilterTimeConstant=0.001  UdotUserProvided=0
  - : PMIOPort  Side=Left
  + : PMIOPort  Port=2  Side=Right
  wires:
  s/1 -> Simulink-PS Converter/1
  connections:
  -/RConn1 -- Controlled Voltage Source/RConn2
  Simulink-PS Converter/RConn1 -- Controlled Voltage Source/RConn1
  Controlled Voltage Source/LConn1 -- +/RConn1

== system PVAndBatteryIntegratedPlantForBlackStart/Battery Inverter/VOC Control/VOC_DE/Current Measurement ==
  Current Sensor : fl_lib/Electrical/Electrical Sensors/Current Sensor
  PS-Simulink Converter : nesl_utility/PS-Simulink Converter  PhysicalDomain=network_engine_domain  SubClassName=ps_output  LeftPortType=input  RightPortType=output  PseudoPeriodic=off  Frequencies=[]  VectorFormat=1-D array  Unit=A  AffineConversion=off
  + : PMIOPort  Side=Left
  - : PMIOPort  Port=2  Side=Right
  i : Outport  VectorParamsAs1DForOutWhenUnconnected=off
  wires:
  PS-Simulink Converter/1 -> i/1
  connections:
  +/RConn1 -- Current Sensor/LConn1
  -/RConn1 -- Current Sensor/RConn2
  PS-Simulink Converter/LConn1 -- Current Sensor/RConn1

== system PVAndBatteryIntegratedPlantForBlackStart/Battery Inverter/VOC Control/VOC_DE/Parallel RLC Branch1 ==
  Inductor : fl_lib/Electrical/Electrical Elements/Inductor  l=L H  r=0 Ohm  g=1e-9 1/Ohm  i_specify=off  i_priority=None  i=0 A  i_nominal_specify=off  i_nominal_value=1  i_nominal_unit=A  v_specify=off  v_priority=None  v=0 V  v_nominal_specify=off  v_nominal_value=1  v_nominal_unit=V  i_L_specify=on  i_L_priority=High  i_L=0 A  i_L_nominal_specify=off  i_L_nominal_value=1  i_L_nominal_unit=A
  + : PMIOPort  Side=Left
  - : PMIOPort  Port=2  Side=Right
  connections:
  -/RConn1 -- Inductor/RConn1
  Inductor/LConn1 -- +/RConn1

== system PVAndBatteryIntegratedPlantForBlackStart/Battery Inverter/VOC Control/VOC_DE/Parallel RLC Branch2 ==
  Capacitor : fl_lib/Electrical/Electrical Elements/Capacitor  c=C F  r=1e-6 Ohm  g=0 1/Ohm  i_specify=off  i_priority=None  i=0 A  i_nominal_specify=off  i_nominal_value=1  i_nominal_unit=A  v_specify=off  v_priority=None  v=0 V  v_nominal_specify=off  v_nominal_value=1  v_nominal_unit=V  vc_specify=on  vc_priority=High  vc=V_voc_1 V  vc_nominal_specify=off  vc_nominal_value=1  vc_nominal_unit=V
  + : PMIOPort  Side=Left
  - : PMIOPort  Port=2  Side=Right
  connections:
  Capacitor/RConn1 -- -/RConn1
  +/RConn1 -- Capacitor/LConn1

== system PVAndBatteryIntegratedPlantForBlackStart/Battery Inverter/VOC Control/VOC_DE/Voltage Measurement ==
  PS-Simulink Converter : nesl_utility/PS-Simulink Converter  PhysicalDomain=network_engine_domain  SubClassName=ps_output  LeftPortType=input  RightPortType=output  PseudoPeriodic=off  Frequencies=[]  VectorFormat=1-D array  Unit=V  AffineConversion=off
  Voltage Sensor : fl_lib/Electrical/Electrical Sensors/Voltage Sensor
  + : PMIOPort  Side=Left
  - : PMIOPort  Port=2  Side=Left
  v : Outport  VectorParamsAs1DForOutWhenUnconnected=off
  wires:
  PS-Simulink Converter/1 -> v/1
  connections:
  PS-Simulink Converter/LConn1 -- Voltage Sensor/RConn1
  -/RConn1 -- Voltage Sensor/RConn2
  +/RConn1 -- Voltage Sensor/LConn1

== system PVAndBatteryIntegratedPlantForBlackStart/PV Inverter /VOC Control/Subsystem/rotate ==
  deltai : Inport
  Demux : Demux  Outputs=2
  Gain : Gain  Gain=-1
  Mux : Mux  Inputs=2
  u : Outport
  wires:
  Demux/1 -> Mux/2
  Gain/1 -> Mux/1
  Demux/2 -> Gain/1
  Mux/1 -> u/1
  deltai/1 -> Demux/1

== system PVAndBatteryIntegratedPlantForBlackStart/PV Inverter /VOC Control/VOC_DE/Controlled Current Source ==
  s : Inport
  Controlled Current Source : fl_lib/Electrical/Electrical Sources/Controlled Current Source
  Simulink-PS Converter : nesl_utility/Simulink-PS Converter  PhysicalDomain=network_engine_domain  SubClassName=ps_input  LeftPortType=input  RightPortType=output  PseudoPeriodic=off  Frequencies=[]  NoiseDistribution=none  NoiseParameters=[]  Unit=1  AffineConversion=off  FilteringAndDerivatives=provide  SimscapeFilterOrder=1  InputFilterTimeConstant=0.001  UdotUserProvided=0
  - : PMIOPort  Side=Left
  + : PMIOPort  Port=2  Side=Right
  wires:
  s/1 -> Simulink-PS Converter/1
  connections:
  Simulink-PS Converter/RConn1 -- Controlled Current Source/RConn1
  Controlled Current Source/RConn2 -- -/RConn1
  Controlled Current Source/LConn1 -- +/RConn1

== system PVAndBatteryIntegratedPlantForBlackStart/PV Inverter /VOC Control/VOC_DE/Controlled Current Source1 ==
  s : Inport
  Controlled Current Source : fl_lib/Electrical/Electrical Sources/Controlled Current Source
  Simulink-PS Converter : nesl_utility/Simulink-PS Converter  PhysicalDomain=network_engine_domain  SubClassName=ps_input  LeftPortType=input  RightPortType=output  PseudoPeriodic=off  Frequencies=[]  NoiseDistribution=none  NoiseParameters=[]  Unit=1  AffineConversion=off  FilteringAndDerivatives=provide  SimscapeFilterOrder=1  InputFilterTimeConstant=0.001  UdotUserProvided=0
  - : PMIOPort  Side=Left
  + : PMIOPort  Port=2  Side=Right
  wires:
  s/1 -> Simulink-PS Converter/1
  connections:
  Simulink-PS Converter/RConn1 -- Controlled Current Source/RConn1
  Controlled Current Source/RConn2 -- -/RConn1
  Controlled Current Source/LConn1 -- +/RConn1

== system PVAndBatteryIntegratedPlantForBlackStart/PV Inverter /VOC Control/VOC_DE/Controlled Voltage Source1 ==
  s : Inport
  Controlled Voltage Source : fl_lib/Electrical/Electrical Sources/Controlled Voltage Source
  Simulink-PS Converter : nesl_utility/Simulink-PS Converter  PhysicalDomain=network_engine_domain  SubClassName=ps_input  LeftPortType=input  RightPortType=output  PseudoPeriodic=off  Frequencies=[]  NoiseDistribution=none  NoiseParameters=[]  Unit=1  AffineConversion=off  FilteringAndDerivatives=provide  SimscapeFilterOrder=1  InputFilterTimeConstant=0.001  UdotUserProvided=0
  - : PMIOPort  Side=Left
  + : PMIOPort  Port=2  Side=Right
  wires:
  s/1 -> Simulink-PS Converter/1
  connections:
  -/RConn1 -- Controlled Voltage Source/RConn2
  Simulink-PS Converter/RConn1 -- Controlled Voltage Source/RConn1
  Controlled Voltage Source/LConn1 -- +/RConn1

== system PVAndBatteryIntegratedPlantForBlackStart/PV Inverter /VOC Control/VOC_DE/Controlled Voltage Source2 ==
  s : Inport
  Controlled Voltage Source : fl_lib/Electrical/Electrical Sources/Controlled Voltage Source
  Simulink-PS Converter : nesl_utility/Simulink-PS Converter  PhysicalDomain=network_engine_domain  SubClassName=ps_input  LeftPortType=input  RightPortType=output  PseudoPeriodic=off  Frequencies=[]  NoiseDistribution=none  NoiseParameters=[]  Unit=1  AffineConversion=off  FilteringAndDerivatives=provide  SimscapeFilterOrder=1  InputFilterTimeConstant=0.001  UdotUserProvided=0
  - : PMIOPort  Side=Left
  + : PMIOPort  Port=2  Side=Right
  wires:
  s/1 -> Simulink-PS Converter/1
  connections:
  -/RConn1 -- Controlled Voltage Source/RConn2
  Simulink-PS Converter/RConn1 -- Controlled Voltage Source/RConn1
  Controlled Voltage Source/LConn1 -- +/RConn1

== system PVAndBatteryIntegratedPlantForBlackStart/PV Inverter /VOC Control/VOC_DE/Current Measurement ==
  Current Sensor : fl_lib/Electrical/Electrical Sensors/Current Sensor
  PS-Simulink Converter : nesl_utility/PS-Simulink Converter  PhysicalDomain=network_engine_domain  SubClassName=ps_output  LeftPortType=input  RightPortType=output  PseudoPeriodic=off  Frequencies=[]  VectorFormat=1-D array  Unit=A  AffineConversion=off
  + : PMIOPort  Side=Left
  - : PMIOPort  Port=2  Side=Right
  i : Outport  VectorParamsAs1DForOutWhenUnconnected=off
  wires:
  PS-Simulink Converter/1 -> i/1
  connections:
  +/RConn1 -- Current Sensor/LConn1
  -/RConn1 -- Current Sensor/RConn2
  PS-Simulink Converter/LConn1 -- Current Sensor/RConn1

== system PVAndBatteryIntegratedPlantForBlackStart/PV Inverter /VOC Control/VOC_DE/Parallel RLC Branch1 ==
  Inductor : fl_lib/Electrical/Electrical Elements/Inductor  l=L H  r=0 Ohm  g=1e-9 1/Ohm  i_specify=off  i_priority=None  i=0 A  i_nominal_specify=off  i_nominal_value=1  i_nominal_unit=A  v_specify=off  v_priority=None  v=0 V  v_nominal_specify=off  v_nominal_value=1  v_nominal_unit=V  i_L_specify=on  i_L_priority=High  i_L=0 A  i_L_nominal_specify=off  i_L_nominal_value=1  i_L_nominal_unit=A
  + : PMIOPort  Side=Left
  - : PMIOPort  Port=2  Side=Right
  connections:
  -/RConn1 -- Inductor/RConn1
  Inductor/LConn1 -- +/RConn1

== system PVAndBatteryIntegratedPlantForBlackStart/PV Inverter /VOC Control/VOC_DE/Parallel RLC Branch2 ==
  Capacitor : fl_lib/Electrical/Electrical Elements/Capacitor  c=C F  r=1e-6 Ohm  g=0 1/Ohm  i_specify=off  i_priority=None  i=0 A  i_nominal_specify=off  i_nominal_value=1  i_nominal_unit=A  v_specify=off  v_priority=None  v=0 V  v_nominal_specify=off  v_nominal_value=1  v_nominal_unit=V  vc_specify=on  vc_priority=High  vc=V_voc_2 V  vc_nominal_specify=off  vc_nominal_value=1  vc_nominal_unit=V
  + : PMIOPort  Side=Left
  - : PMIOPort  Port=2  Side=Right
  connections:
  Capacitor/RConn1 -- -/RConn1
  +/RConn1 -- Capacitor/LConn1

== system PVAndBatteryIntegratedPlantForBlackStart/PV Inverter /VOC Control/VOC_DE/Voltage Measurement ==
  PS-Simulink Converter : nesl_utility/PS-Simulink Converter  PhysicalDomain=network_engine_domain  SubClassName=ps_output  LeftPortType=input  RightPortType=output  PseudoPeriodic=off  Frequencies=[]  VectorFormat=1-D array  Unit=V  AffineConversion=off
  Voltage Sensor : fl_lib/Electrical/Electrical Sensors/Voltage Sensor
  + : PMIOPort  Side=Left
  - : PMIOPort  Port=2  Side=Left
  v : Outport  VectorParamsAs1DForOutWhenUnconnected=off
  wires:
  PS-Simulink Converter/1 -> v/1
  connections:
  PS-Simulink Converter/LConn1 -- Voltage Sensor/RConn1
  -/RConn1 -- Voltage Sensor/RConn2
  +/RConn1 -- Voltage Sensor/LConn1
